simulink model "sim_main_esb_3"  (R2018b)
settings: Solver=VariableStepAuto  StartTime=0.0  StopTime=1  RelTol=1e-3
values from neighbouring files (symbols this model uses):
  A = 0.914    [KALMAN.m]    (also in main_cntl.m = eval(A_eq); main_sys.m = double(A_lin); main_sys_klm.m = double(A_lin); main_tf_0.m = A)
  A_lin = subs(A_eq)    [main_sys.m]    (also in main_sys_klm.m; main_tf_10.m; main_tf_11.m; main_tf_12.m)
  B = 0.25    [KALMAN.m]    (also in main_cntl.m = eval(B_eq); main_sys.m = double(B_lin); main_sys_klm.m = double(B_lin); main_tf_1.m = eval(B))
  B_lin = subs(B_eq)    [main_sys.m]    (also in main_sys_klm.m; main_tf_10.m; main_tf_11.m; main_tf_12.m)
  bm = 0.4e-3    (= 0.0004)    [main_cntl.m]    (also in main_sys.m = 0.00047698; main_sys_klm.m = 0.00047698; main_tf_1.m; main_tf_10.m = 0.00047698)
  C = 0.344    [KALMAN.m]    (also in main_sys.m = double( subs( C) ); main_sys_klm.m = double( subs( C) ); main_tf_0.m = [ 0 , 0  , Ks , ds , -Ks , -ds, 0 ]; main_tf_1.m = C_mes)
  C_lin = subs(C_eq)    [main_sys.m]    (also in main_sys_klm.m; main_tf_1.m = C; main_tf_10.m; main_tf_11.m)
  D_lin = zeros(1,2)    [main_sys.m]    (also in main_sys_klm.m; main_tf_10.m; main_tf_11.m; main_tf_12.m)
  dg = 0.65    [main_cntl.m]    (also in main_sys.m; main_sys_klm.m; main_tf_1.m; main_tf_10.m)
  dgs = 6    [main_cntl.m]    (also in main_sys.m; main_sys_klm.m; main_tf_1.m; main_tf_10.m)
  dh = 0.75    [main_cntl.m]    (also in main_sys.m; main_sys_klm.m; main_tf_1.m; main_tf_10.m)
  dhs = 0    [main_cntl.m]    (also in main_sys.m; main_sys_klm.m; main_tf_1.m; main_tf_10.m)
  ds = 0.001    [main_cntl.m]    (also in main_sys.m = 0; main_sys_klm.m = 0; main_tf_1.m = 0; main_tf_10.m = 0)
  J_act = [0.000306 +  0.28200e-04]    [main_cntl.m]    (also in main_sys.m; main_sys_klm.m; main_tf_1.m; main_tf_10.m)
  Jh = 5.02    [main_cntl.m]    (also in main_sys.m; main_sys_klm.m; main_tf_1.m; main_tf_10.m)
  Js_ext = 9.58e-4    (= 0.000958)    [main_cntl.m]    (also in main_sys.m; main_sys_klm.m; main_tf_1.m; main_tf_10.m)
  Js_int = 1.1e-4    (= 0.00011)    [main_cntl.m]    (also in main_sys.m; main_sys_klm.m; main_tf_1.m; main_tf_10.m)
  Kg = 2.7e4    (= 27000)    [main_cntl.m]    (also in main_sys.m; main_sys_klm.m; main_tf_1.m; main_tf_10.m)
  Kh = 1125    [main_cntl.m]    (also in main_sys.m; main_sys_klm.m; main_tf_1.m; main_tf_10.m)
  Ks = 8.1853e4*1.4    (= 114594.2)    [main_cntl.m]    (also in main_sys.m; main_sys_klm.m; main_tf_1.m; main_tf_10.m)
  Q = 0.01^2    (= 0.0001)    [KALMAN.m]    (also in main_cntl.m = 2e10.*eye(6,6); main_sys.m = 1e15.*eye(8,8); main_sys_klm.m = 1e1.*eye(8,8); main_tf_1.m = 1)
  R = 0.1^2    (= 0.01)    [KALMAN.m]    (also in main_cntl.m = 1; main_sys.m = 1; main_sys_klm.m = 1; main_tf_1.m = .5*diag(ones(1,1)))
  rg = 160    [main_cntl.m]    (also in main_sys.m; main_sys_klm.m; main_tf_1.m; main_tf_10.m)
  Ts = -1    [main_cntl.m]    (also in main_sys.m; main_sys_klm.m; main_tf_1.m; main_tf_10.m)
  Vel_mot_nom = 263    [main_cntl.m]    (also in main_sys.m; main_sys_klm.m; main_tf_1.m; main_tf_10.m)
settings Model: Creator=eshojaei  LastModifiedBy=eshojaei

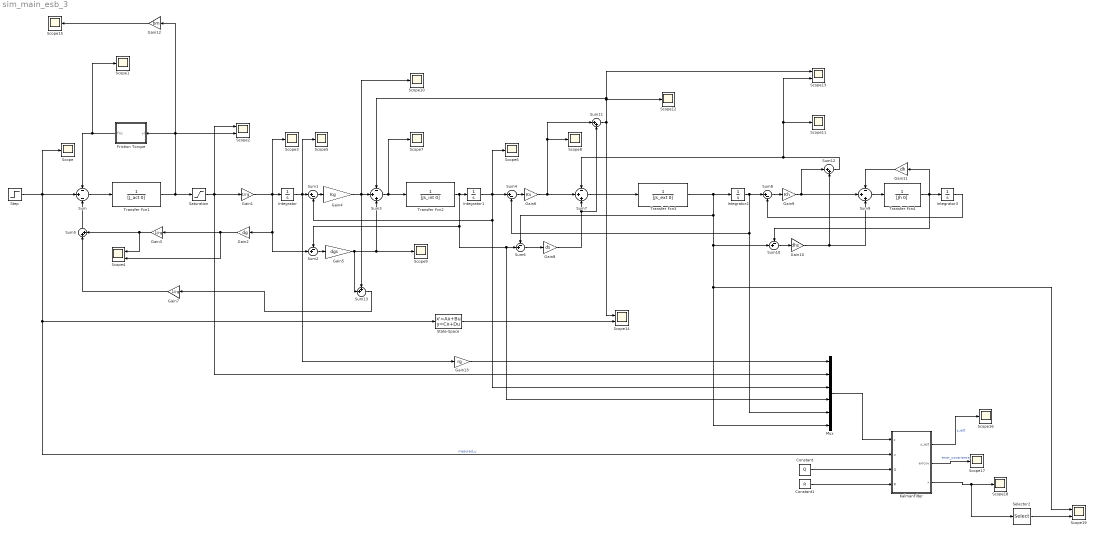
== system sim_main_esb_3 ==
  Constant : Constant  Value=Q  SampleTime=Ts
  Constant1 : Constant  Value=R  SampleTime=Ts
  Friction Torque : MATLAB Function  TreatAsAtomicUnit=on
  Gain1 : Gain  Gain=1/rg
  Gain10 : Gain  Gain=dhs
  Gain11 : Gain  Gain=dh
  Gain12 : Gain  Gain=bm
  Gain13 : Gain  Gain=rg
  Gain2 : Gain  Gain=dg
  Gain3 : Gain  Gain=1/rg
  Gain4 : Gain  Gain=Kg
  Gain5 : Gain  Gain=dgs
  Gain6 : Gain  Gain=Ks
  Gain7 : Gain  Gain=1/rg
  Gain8 : Gain  Gain=ds
  Gain9 : Gain  Gain=Kh
  Integrator{,1..3} (4 alike) : Integrator
  KalmanFilter : Subsystem
  Mux : Mux  Inputs=6
  Saturation : Saturate  UpperLimit=Vel_mot_nom  LowerLimit=-Vel_mot_nom
  Scope{,1,3,5..12,15..18} (15 alike) : Scope
  Scope{2,4,13..14,19} (5 alike) : Scope  NumInputPorts=2
  Selector2 : Selector  InputPortWidth=8  IndexOptions=Index vector (dialog)  Indices=[6]  OutputSizes=1
  State-Space : StateSpace  A=A_lin  B=B_lin  C=C_lin  D=D_lin  InitialCondition=0
  Step : Step  Time=.1  After=.04  SampleTime=0
  Sum : Sum  Inputs=-|+|-
  Sum1 : Sum  Inputs=|+-
  Sum10 : Sum  Inputs=-+|
  Sum11 : Sum  Inputs=|++
  Sum12 : Sum  Inputs=|++
  Sum13 : Sum  Inputs=++|
  Sum2 : Sum  Inputs=-+|
  Sum3 : Sum  Inputs=-++
  Sum4 : Sum  Inputs=|+-
  Sum5 : Sum  Inputs=|++
  Sum6 : Sum  Inputs=-+|
  Sum7 : Sum  Inputs=-++
  Sum8 : Sum  Inputs=|+-
  Sum9 : Sum  Inputs=-++
  Transfer Fcn1 : TransferFcn  Denominator=[J_act 0]
  Transfer Fcn2 : TransferFcn  Denominator=[Js_int 0]
  Transfer Fcn3 : TransferFcn  Denominator=[Js_ext 0]
  Transfer Fcn4 : TransferFcn  Denominator=[Jh 0]
  wires:
  Gain6/1 -> Sum7/2, Sum11/1, Scope8/1
  Sum/1 -> Transfer Fcn1/1
  Transfer Fcn1/1 -> Saturation/1, Gain12/1, Friction Torque/1(vl), Scope2/2
  Gain4/1 -> Sum3/2, Sum13/1, Scope10/1
  Transfer Fcn2/1 -> Mux/4, Sum6/2, Sum2/1, Integrator1/1
  Gain7/1 -> Sum5/1
  Integrator/1 -> Gain13/1, Sum1/1, Scope5/1
  Sum1/1 -> Gain4/1
  Transfer Fcn3/1 -> Integrator2/1, Sum10/2, Scope19/1, Mux/6, Sum6/1
  Sum5/1 -> Sum/3
  Sum3/1 -> Transfer Fcn2/1, Scope7/1
  Gain5/1 -> Sum3/3, Scope9/1, Sum13/2
  Gain2/1 -> Scope4/2, Gain3/1
  Gain1/1 -> Scope3/1, Integrator/1, Sum2/2, Gain2/1
  Gain3/1 -> Sum5/2, Scope4/1
  Sum2/1 -> Gain5/1
  Sum4/1 -> Gain6/1
  Sum6/1 -> Gain8/1
  Gain8/1 -> Sum11/2, Sum7/3
  Sum7/1 -> Transfer Fcn3/1
  Sum8/1 -> Gain9/1
  Gain9/1 -> Sum12/1, Sum9/2
  Sum9/1 -> Transfer Fcn4/1
  Transfer Fcn4/1 -> Gain11/1, Sum10/1, Integrator3/1
  Integrator3/1 -> Sum8/2
  Gain10/1 -> Sum12/2, Sum9/3
  Sum10/1 -> Gain10/1
  Gain11/1 -> Sum9/1
  Sum11/1 -> Scope13/1, Sum3/1, Scope12/1, Scope14/1
  Sum12/1 -> Scope11/1, Scope13/2, Sum7/1
  Gain12/1 -> Scope15/1
  Sum13/1 -> Gain7/1
  Friction Torque/1(fric) -> Sum/1, Scope1/1
  State-Space/1 -> Scope14/2
  Step/1 -> Sum/2, State-Space/1, KalmanFilter/2(u), Scope/1  "mesured_u"
  Gain13/1 -> Mux/1
  Integrator1/1 -> Sum4/1, Scope6/1, Mux/3, Sum1/2
  Mux/1 -> KalmanFilter/1(z)
  Constant/1 -> KalmanFilter/3(Q)
  Constant1/1 -> KalmanFilter/4(R)
  KalmanFilter/1(y_est) -> Scope16/1  "y_est"
  KalmanFilter/2(errcov) -> Scope17/1  "error_covariance"
  KalmanFilter/3(x) -> Selector2/1, Scope18/1
  Saturation/1 -> Mux/2, Gain1/1, Scope2/1
  Selector2/1 -> Scope19/2
  Integrator2/1 -> Sum8/1, Mux/5, Sum4/2

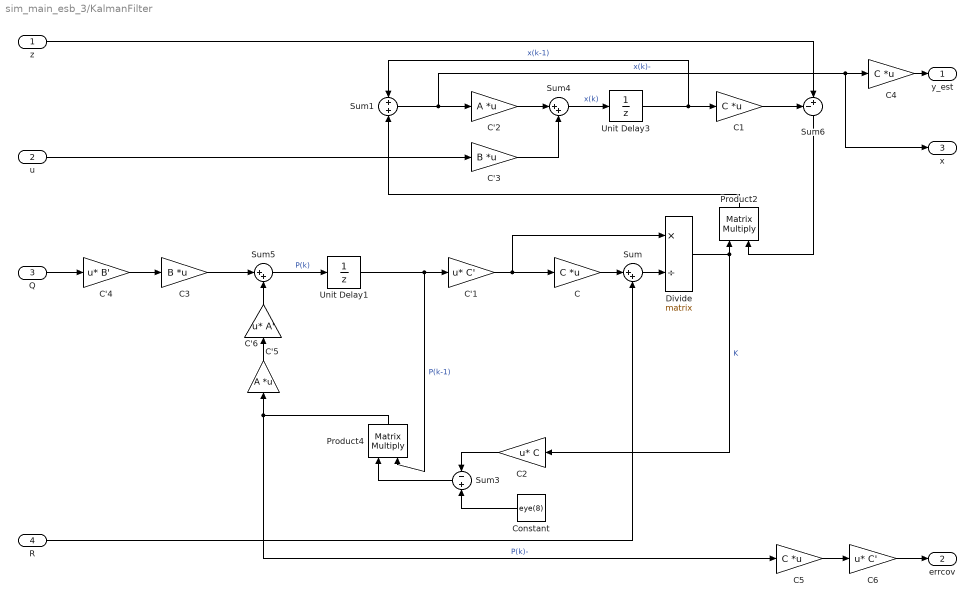
== system sim_main_esb_3/KalmanFilter ==
  z : Inport
  u : Inport  Port=2
  Q : Inport  Port=3
  R : Inport  Port=4
  C{,1,4..5} (4 alike) : Gain  Gain=C  Multiplication=Matrix(K*u)
  C'1 : Gain  Gain=C'  Multiplication=Matrix(u*K)
  C'2 : Gain  Gain=A  Multiplication=Matrix(K*u)
  C'3 : Gain  Gain=B  Multiplication=Matrix(K*u)
  C'4 : Gain  Gain=B'  Multiplication=Matrix(u*K)
  C'5 : Gain  Gain=A  Multiplication=Matrix(K*u)
  C'6 : Gain  Gain=A'  Multiplication=Matrix(u*K)
  C2 : Gain  Gain=C  Multiplication=Matrix(u*K)
  C3 : Gain  Gain=B  Multiplication=Matrix(K*u)
  C6 : Gain  Gain=C'  Multiplication=Matrix(u*K)
  Constant : Constant  Value=eye(8)
  Divide : Product  Inputs=*/  Multiplication=Matrix(*)
  Product2 : Product  Multiplication=Matrix(*)  RndMeth=Zero
  Product4 : Product  Multiplication=Matrix(*)  RndMeth=Zero
  Sum : Sum  Inputs=|++
  Sum1 : Sum
  Sum3 : Sum  Inputs=-+
  Sum4 : Sum  Inputs=|++
  Sum5 : Sum  Inputs=|++
  Sum6 : Sum  Inputs=-+|
  Unit Delay1 : UnitDelay  InitialCondition=zeros(8,8)  SampleTime=Ts
  Unit Delay3 : UnitDelay  InitialCondition=zeros(8,1)  SampleTime=Ts
  y_est : Outport
  errcov : Outport  Port=2
  x : Outport  Port=3
  wires:
  Unit Delay3/1 -> Sum1/1, C1/1  "x(k-1)"
  Unit Delay1/1 -> C'1/1, Product4/2  "P(k-1)"
  R/1 -> Sum/2
  Sum/1 -> Divide/2
  Divide/1 -> C2/1, Product2/1  "K"
  C1/1 -> Sum6/1
  z/1 -> Sum6/2
  Product2/1 -> Sum1/2
  C'1/1 -> C/1, Divide/1
  C/1 -> Sum/1
  Constant/1 -> Sum3/2
  C2/1 -> Sum3/1
  Product4/1 -> C'5/1, C5/1  "P(k)-"
  Sum1/1 -> C'2/1, C4/1, x/1  "x(k)-"
  u/1 -> C'3/1
  Sum4/1 -> Unit Delay3/1  "x(k)"
  C'2/1 -> Sum4/1
  C'3/1 -> Sum4/2
  C'4/1 -> C3/1
  Q/1 -> C'4/1
  C3/1 -> Sum5/1
  C'5/1 -> C'6/1
  C'6/1 -> Sum5/2
  Sum5/1 -> Unit Delay1/1  "P(k)"
  C5/1 -> C6/1
  C4/1 -> y_est/1
  C6/1 -> errcov/1
  Sum6/1 -> Product2/2
  Sum3/1 -> Product4/1

== matlab function sim_main_esb_3/Friction Torque ==
  data: vl input; fric output
function fric = fcn(vl)

    
   fric = (5981672325465929*vl)/147573952589676412928 + (7059617857129123*tanh((6072588977179245*vl)/36028797018963968))/144115188075855872 + (2558104915892175*tanh((5176012883402097*vl)/576460752303423488))/72057594037927936;
